simulink model "Dynamics_v2_temp"  (R2021b)
settings: Solver=VariableStepAuto  StartTime=0.0  StopTime=10.0  RelTol=1e-3
InitFcn:
  | % ************** Initiate forces
  | % f0=[0;0;0;0;0;0];
  | % f0=[0;0;0;0;0;0;0];
  | f_0=[0;0;0];
  | f_m=[0;0];
  | f_e=[0;0;0;0;0;0];
  | % ************** Initiate states
  | q_m=[0;0];
  | q_dot_m=[0;0];
  | P=[0;0;0];
  | V_I0=[0;0;0];
  | % ************** Load main
  | %run(Main.m)
values from neighbouring files (symbols this model uses):
  diag_M = diagonalize(M_frak0, M_frak)    [Create_Robot.m]    (also in Main.m; diagonalize.m = zeros(6*(n+1),6*(n+1)); test_C_Main.m)
  iota0 = [1 0 0; 0 1 0;zeros(3,3);0 0 1]    [Create_Robot.m]    (also in Main.m = eye(6,6); test_C_Main.m)
  M_curly = zeros(n,6,6)    [M_curly.m]
  mu = zeros(6,1)'    [Create_Robot.m]    (also in Main.m; test_C_Main.m)
  Xi_m_matrix = zeros(6*n,n)    [Create_Robot.m]    (also in Main.m; test_C_Main.m)
undefined symbols (not defined in the file or in its folder): Ad_gm_inv, g_bar, M_curly0, Xi_m
(part 2 of 2)

== matlab function Dynamics_v2_temp/Inverse Dynamics/Internal Dynamics/N_hat/N_hat ==
  data: N_hat output; q_m input; q_dot_m input; A input; V input; P input; M0_partial input; A_partial input; iota0 input
function N_hat = N_hat(q_m,q_dot_m,A,V,P,M0_partial, A_partial, iota0)
% Calculates the N_hat_m matrix from base pose and arm joint angles

n=length(q_m);
b=length(V);

%Form N_hat from equation 19 of ACC paper
N_temp1=zeros(n,b); N_temp2=zeros(n,b); N_temp3=zeros(n,b);

for i=1:n
    N_temp1=N_temp1+transpose(squeeze(A_partial(1:b,1:n,i)).*q_dot_m(i)); % transpose of (bxn times 1x1)
    N_temp2(i,1:b)=transpose(q_dot_m)*transpose(squeeze(A_partial(1:b,1:n,i))); %1xn times nxb
    N_temp3(i,1:b)=0.5*transpose(P)*squeeze(M0_partial(1:b,1:b,i)); % 1xb times bxb
end

N_hat=transpose(A)*transpose(adjoint_low(V,iota0))*P-N_temp1*P+N_temp2*P+N_temp3*P;

== matlab function Dynamics_v2_temp/time-dependent variables' calculations/  ==
  data: q_m input; L0 output; Lm0 output; Lm output; Xi_m input
function [L0,Lm0,Lm] =L_calculator(q_m,Xi_m)
% Calculates the time-dependent L matrix
n=length(q_m);
L=zeros(6*(n+1),6*(n+1));
% Compute M_frak for ith body
% Calculate L matrix
for i=1:n+1
    for j=1:n+1
        if i>j
            Ad_temp=eye(6);
            for k=j:i-1
                Ad_temp=Adjoint(g_Matrix(-Xi_m(:,k),q_m(k)))*Ad_temp;
            end
            L(6*(i-1)+1:6*(i-1)+6,6*(j-1)+1:6*(j-1)+6)=Ad_temp;
        elseif i==j
            L(6*(i-1)+1:6*(i-1)+6,6*(j-1)+1:6*(j-1)+6)=eye(6);
        elseif i<j
            L(6*(i-1)+1:6*(i-1)+6,6*(j-1)+1:6*(j-1)+6)=zeros(6);
        end
    end
end

L0=L(1:6,1:6);
Lm0=L(7:end,1:6);
Lm=L(7:end,7:end);

end

== matlab function Dynamics_v2_temp/time-dependent variables' calculations/MATLAB Function ==
  data: M0 input; M0m input; A output
function A=A_connection(M0,M0m)
% Compute the connection A from mass properties

A=M0\M0m;

== matlab function Dynamics_v2_temp/time-dependent variables' calculations/Jacobian End Effector/Jacobian_ee ==
  data: J_e0 output; q_m input; Xi_m input; J_em output; V input; iota0 input; g_0e input
function [J_e0, J_em] = Jacobian_end_effector(q_m,Xi_m,V,iota0, g_0e)
% Calculates the body Velocity of end-effector from arm joint angles

n=length(q_m);
b=length(V);

% Initiate
J=zeros(6,b+n);
% Jm=zeros(6,robot.n);

% Vehicle portion
J0=iota0;
J(1:6,1:b)=J0;

% ____________ Manipulator Jacobian _____________ %

% Initiate
j=1;
Jm=zeros(6,n);

Jm(:,j)=Xi_m(:,j);
for j=2:n %Iterate through all joints
    temp=eye(6);
    for i=1:j-1
        temp=temp*Adjoint(g_Matrix(Xi_m(:,i),q_m(i)));
    end
    Jm(:,j)=temp*Xi_m(:,j);
end

J(:,b+1:b+n)=Jm;

J_ee0=Adjoint(g_0e)\J;
% J_eeI=Adjoint(g_I0)*J_ee0; % transform to inertia

J_e0=J_ee0(1:6,1:b);
J_em=J_ee0(1:6,b+1:end);

end

== matlab function Dynamics_v2_temp/Simulink Function11/MATLAB Function ==
  data: J_e0 output; q_m input; Xi_m input; J_em output
function [J_e0, J_em] = Jacobian_end_effector( q_m,Xi_m)
% Calculates the body Velocity of end-effector from base pose and arm joint angles

% Compute the geometric Jacobian of the point rp
%   	rp  point of interest in inertial frame 
%       i   link number

n=length(q_m);

% Initiate
J=zeros(6,6 + n);
% Jm=zeros(6,n);

% Vehicle portion
J0=eye(6,6);
J(1:6,1:6)=J0;

% ____________ Manipulator Jacobian _____________ %

% Initiate
j=1;
Jm=zeros(6,n);

Jm(1:6,j)=Xi_m(1:6,j);
for j=2:n %Iterate through all joints
    for i=1:j-1
        temp=Adjoint(expm(skewsym(Xi_m(i))*q_m(i)));
    end
    Jm(1:6,j)=temp*Xi_m(j);
end


J_ee0=[J0 Jm(1:6,1:n)];
% J_eeI=Adjoint(g_I0)*J_ee0; % transform to inertia

J_e0=J_ee0(1:6,1:6);
J_em=J_ee0(1:6,7:n);

end

== matlab function Dynamics_v2_temp/Inverse Dynamics/Internal Dynamics/C_hat/Lm_partials/Lmpartial ==
  data: q_m input; Lm_partial output; Xi_m input; iota0 input
function Lm_partial = Lm_partial(q_m,Xi_m,iota0)
% Calculates the C_hat_m matrix from base pose and arm joint angles

n=length(q_m);

% Find partial of Lm0 to joint angles
Lm_partial=zeros(6*n,6*n,n); % 6nx6xn
for i=1:n
    for j=1:n
        for k=1:n
            Lm_partial(6*(j-1)+1:6*j,6*(k-1)+1:6*k,i)=Ad_partial(j,k,i,Xi_m,q_m,iota0); % equation 114 of TRO paper
            if j==k
                Lm_partial(6*(j-1)+1:6*j,6*(k-1)+1:6*k,i)=eye(6,6);
            end
        end
    end
end

== matlab function Dynamics_v2_temp/Inverse Dynamics/Internal Dynamics/C_hat/M_partials/ M0partial ==
  data: q_m input; M0_partial output; Lm0 input; V input; iota0 input; diag_Mm input; Lm0_partial input
function M0_partial = M0_partial(q_m,Lm0,V,iota0,diag_Mm,Lm0_partial)
% Calculates the C_hat_m matrix from base pose and arm joint angles

n=length(q_m);
b=length(V);

% Find partial of M0 to joint angles
M0_partial=zeros(b,b,n); %initiate
for i=1:n
    M0_partial(1:b,1:b,i)= iota0'*(transpose(Lm0_partial(1:6*n,1:6,i))*diag_Mm*Lm0+transpose(Lm0)*diag_Mm*Lm0_partial(1:6*n,1:6,i))*iota0; %6x6 %equation 117 of TRO
end

== matlab function Dynamics_v2_temp/Inverse Dynamics/Internal Dynamics/C_hat/M_partials/M0mpartial ==
  data: q_m input; M0m_partial output; V input; Lm0 input; iota0 input; diag_Mm input; Lm0_partial input; Lm_partial input
function M0m_partial = M0m_partial(q_m,V,Lm0,iota0,diag_Mm,Lm0_partial,Lm_partial)
% Calculates the C_hat_m matrix from base pose and arm joint angles

n=length(q_m);
b=length(V);

% Find partial of M0m to joint angles
M0m_partial=zeros(b,n,n);
for i=1:n
    M0m_partial(1:b,1:n,i)= iota0'*((transpose(squeeze(Lm0_partial(1:6*n,1:6,i)))*diag_Mm*Lm0+transpose(Lm0)*diag_Mm*Lm_partial(1:6*n,1:6*n,i)))*Xi_m_matrix; % equation 118 of TRO paper
end

== matlab function Dynamics_v2_temp/time-dependent variables' calculations/Mass Matrix Blocks/MATLAB Function ==
  data: diag_M input; m0_frak output; m_diag output
function [m0_frak,m_diag]=m_frak_decomp(diag_M)
% Compute the Mass Matrix of the multibody system.
%   Output:
%   M0      Spacecraft mass matrix 
%   M0m
%   Mm      Manipulator mass matrix

%n=length(q_m);

m0_frak=diag_M(1:6,1:6);
m_diag=diag_M(7:end,7:end);

== matlab function Dynamics_v2_temp/Inverse Dynamics/Internal Dynamics/C_hat/MATLAB Function4 ==
  data: q_m input; A_partial output; M0 input; M0m input; V input; M0_partial input; M0m_partial input
function A_partial = A_partial(q_m,M0,M0m,V,M0_partial,M0m_partial)
% Calculates the C_hat_m matrix from base pose and arm joint angles

n=length(q_m);
b=length(V);

% Find partial of connection A to each joint angle
A_partial=zeros(b,n,n);

temp1=zeros(b,n);
temp2=zeros(b,n);
temp3=zeros(b,n);

for i=1:n
    temp1=M0\M0_partial(1:b,1:b,i);
    temp2=M0\M0m;
    temp3=M0\M0m_partial(1:b,1:n,i);
    A_partial(1:b,1:n,i)=temp1*temp2+temp3; % Equation 122
end

== matlab function Dynamics_v2_temp/Inverse Dynamics/Internal Dynamics/C_hat/M_partials/Mmpartial ==
  data: q_m input; Mm_partial output; Xi_m_Matrix input; Lm input; diag_Mm input; Lm_partial input
function Mm_partial = Mm_partial(q_m,Xi_m_Matrix,Lm,diag_Mm,Lm_partial)
% Calculates the C_hat_m matrix from base pose and arm joint angles

n=length(q_m);

% find the non-generalized arm mass matrix'x derivative to joint angles
Mm_partial=zeros(n,n,n);
for i=1:n
    Mm_partial(1:n,1:n,i)=transpose(Xi_m_Matrix)*(transpose(Lm_partial(1:6*n,1:6*n,i))*diag_Mm*Lm + ...
        transpose(Lm)*diag_Mm*Lm_partial(1:6*n,1:6*n,i))*Xi_m_Matrix; %calcualte the derivative of not-augmented arm mass matrix from equation 120 of TRO paper
end

== matlab function Dynamics_v2_temp/Inverse Dynamics/Internal Dynamics/C_hat/MATLAB Function6 ==
  data: q_m input; AMA_partial output; M0 input; A input; V input; M0_partial input; A_partial input
function AMA_partial = AMA_partial(q_m,M0,A,V,M0_partial,A_partial)
% Calculates the C_hat_m matrix from base pose and arm joint angles

n=length(q_m);
b=length(V);

% find the temp intermediate term
AMA_partial=zeros(n,n,n);
for i=1:n
    AMA_partial(1:n,1:n,i)=transpose(A_partial(1:b,1:n,i))*M0*A+transpose(A)*M0_partial(1:b,1:b,i)*A+transpose(A)*M0*A_partial(1:b,1:n,i); %calcualte the derivative of not-augmented arm mass matrix from equation 121 of TRO paper
end

== matlab function Dynamics_v2_temp/Inverse Dynamics/Internal Dynamics/C_hat/MATLAB Function7 ==
  data: q_m input; Mm_hat_partial output; Mm_partial input; AMA_partial input
function Mm_hat_partial = Mm_hat_partial(q_m, Mm_partial, AMA_partial)
% Calculates the C_hat_m matrix from base pose and arm joint angles

n=length(q_m);

% find the generalized arm mass matrix'x derivative to joint angles
Mm_hat_partial=zeros(n,n,n);
for i=1:n
    Mm_hat_partial(1:n,1:n,i)=Mm_partial(1:n,1:n,i)-AMA_partial(1:n,1:n,i); %calcualte the derivative of augmented arm mass matrix from equation 119 of TRO paper
end

== matlab function Dynamics_v2_temp/Simulink Function12/MATLAB Function ==
  data: M_frak0 output; M_curly0 input; M_curly input; Ad_gm_inv input; M_frak output
function [M_frak0,M_frak] =M_frak(M_curly0,M_curly,Ad_gm_inv)
% Compute M_frak for ith body

M_frak0=M_curly0;
M_frak=zeros(length(squeeze(M_curly(:,1,1))),6,6);

% Calculate M_frak
for i=1:length(squeeze(M_curly(:,1,1)))
%     Adi_inv=inverse(Adjoint());
    M_frak(i,:,:)=transpose(Ad_gm_inv(:,:,i))*squeeze(M_curly(i,:,:))*Ad_gm_inv(:,:,i);
end

== matlab function Dynamics_v2_temp/time-dependent variables' calculations/V_I0 ==
  data: P input; A_connection input; q_dot_m input; M0 input; V_I0 output
function V_I0=V_I0(P,A_connection,q_dot_m,M0)
% Find the spaccecraft velocity V_I0
% M0_inv=inv(M0);
% temp=P-transpose(A_connection)*q_dot_m;
V_I0=M0\P-A_connection*q_dot_m;

== matlab function Dynamics_v2_temp/Differential Kinematics/MATLAB Function ==
  data: V_Ie output; q_dot_m input; J_e0 input; J_em input; V_I0 input
function V_Ie = Differential_Kinematics(q_dot_m, J_e0, J_em,  V_I0)
% Calculates the body Velocity of end-effector from base pose and arm joint angles
% Using equation 25 of ACC paper

% Calculate the mass matrix at this configuration
% [M0 M0m Mm]=Mass_Matrix(q_m);

% A_connection=inverse(M0)*M0m;

% Find V_I0 from the known total momentum and joint velocities
% V_I0=inverse(M0)*transpose(Adjoint(g_I0))*mu-A_connection*q_dot_m;

% Find the end effector boy velocity 
V_Ie=[J_e0 J_em]*[V_I0;q_dot_m];

== matlab function Dynamics_v2_temp/Simulink Function12/MATLAB Function1 ==
  data: M_frak0 input; M_frak input; diag_M output
function diag_M =diagonalize(M_frak0, M_frak)
% Compute M_frak for ith body
n=length(M_frak(:,1,1));

% Initiate
diag_M=zeros(6*(n+1),6*(n+1));

diag_M(1:6,1:6)=M_frak0;

% Calculate diag{M_frak}
for i=2:(n+1)
    diag_M(6*(i-1)+1:6*i,6*(i-1)+1:6*i)=M_frak(i-1,:,:);
end

end

== matlab function Dynamics_v2_temp/Simulink Function2/Mass_Matrix_Blocks1 ==
  data: I0 input; Im input; m0 input; mm input; M0 output; q_m input; M0m output; Mm output; Xi_m input
function [M0,M0m,Mm]=Mass_Matrix(I0,Im,m0,mm,q_m,Xi_m)
% Compute the Mass Matrix of the multibody system.
%   Output:
%   M0      Spacecraft mass matrix 
%   M0m
%   Mm      Manipulator mass matrix

n=length(q_m);

%Initiate
Mm=zeros(6,6,n,'like',I0);

% Calculate L matrix
for i=1:n
    for j=1:n
        if i>j
            Ad_temp=eye(6);
            for k=i:j
                Ad_temp=Ad_temp*Adjoint(g_matrix(-Xi_m(k),q_m(k)))
            end
            L(6*(i-1)+1:6*(i-1)+6,6*(j-1)+1:6*(j-1)+6)=Ad_temp;
        elseif i==j
            L(6*(i-1)+1:6*(i-1)+6,6*(j-1)+1:6*(j-1)+6)=zeros(6);
        elseif i<j
            L(6*(i-1)+1:6*(i-1)+6,6*(j-1)+1:6*(j-1)+6)=zeros(6);
        end
    end
end

%Backwards recursion
for i=n:-1:1
    %Initialize M 
    Mm(1:6,1:6,i)=[Im(1:3,1:3,i),zeros(3,3);zeros(3,3),mm(i)*eye(3)];
    for j=1:n-i
        Mm(1:6,1:6,i)=Mm_tilde(1:6,1:6,i)+Tij(1:6,1:6,i+j,i)'*Mm(1:6,1:6,i+j)*Tij(1:6,1:6,i+j,i);
        % Conjugation of the Inertia matrix by the translation matrix corresponding to CG
    end
end

% Spacecraft M tilde
M0=[I0,zeros(3,3);zeros(3,3),m0*eye(3)];
for j=1:n
    M0=M0+Ti0(1:6,1:6,j)'*Mm(1:6,1:6,j)*Ti0(1:6,1:6,j);
end


end

== matlab function Dynamics_v2_temp/Simulink Function/MATLAB Function ==
  data: g_I0 input; g_Ie output; q_m input; Xi_m input; g_bar input
function g_Ie = Forward_Kinematics(g_I0, q_m,Xi_m,g_bar)
% Calculates the absolute pose of end-effector from base pose and arm joint angles

% Initiate
g_Ie=g_I0; %the pose of the spacecraft

n=length(q_m);

for i=0:length(q_m)-1
    g_Ie=g_Ie*expm(skewsym(Xi_m(1:6,i))*q_m(i)); % the effect of the motion induced by each joint
end

g_Ie=g_Ie*g_bar(1:4,1:4,end); %multiply by the initial pose of the last link (wrist)

== matlab function Dynamics_v2_temp/Simulink Function2/Mass Matrix Blocks/MATLAB Function ==
  data: diag_M input; m0_frak output; m_diag output
function [m0_frak,m_diag]=m_frak_decomp(diag_M)
% Compute the Mass Matrix of the multibody system.
%   Output:
%   M0      Spacecraft mass matrix 
%   M0m
%   Mm      Manipulator mass matrix

%n=length(q_m);

m0_frak=diag_M(1:6,1:6);
m_diag=diag_M(7:end,7:end);
